simulink model "gm_whdlOFDMTx"  (R2022b)
settings: Solver=FixedStepDiscrete  StartTime=0.0  StopTime=0  RelTol=1e-3
model workspace (MATLAB code in the model file):
  | config = whdlexamples.OFDMTxParameters();
  | fftLen = config.fftLen;
  | subC = config.subC;
  | cpLen = config.cpLen;
  | fs = config.fs;
  | NSS = config.NSS;
  | NRS = config.NRS;
  | NHeader = config.NHeader;
  | NData = config.NData;
  | NSymPerF = config.NSymPerF;
  | ssSymbol = config.ssSymbol;
  | rsSymbol = config.rsSymbol;
  | NHeaderBits = config.NHeaderBits;
  | headerCRCBool = config.headerCRCBool;
  | headerConvK = config.headerConvK;
  | headerConvCode = config.headerConvCode;
  | pilotValPerSym = config.pilotValPerSym;
  | pilotLen = config.pilotLen;
  | dataCRCPoly = config.dataCRCPoly;
  | dataCRCBool = config.dataCRCBool;
  | dataCRCLen = config.dataCRCLen;
  | dataConvK = config.dataConvK;
  | dataConvCode = config.dataConvCode;
  | scramInit = config.scramInit;
  | firCoeff = config.firCoeff;
  | rateFac1 = config.rateFac1;
  | rateFac2 = config.rateFac2;
  | headerLat = config.headerLat;
  | headerTime = config.headerTime;
  | preambleInd = config.preambleInd;
  | headerDataInd = config.headerDataInd;
  | trBlkSize = config.trBlkSize;
  | randOFDM = config.randOFDM;
  | headerIntrlvMaxBlkSize = config.headerIntrlvMaxBlkSize;
  | headerIntrlvNColumns   = config.headerIntrlvNColumns;
  | dataIntrlvMaxBlkSize   = config.dataIntrlvMaxBlkSize;
  | dataIntrlvNColumns     = config.dataIntrlvNColumns;
  | clear config
libraries: hdlsllib x49, simulink x22, dspsigops x11, whdlmod x3, whdledac x3, whdlutilities x2, commhdlcrc x2, dsphdlfiltering2 x1
(part 2 of 4)

== system gm_whdlOFDMTx/Frame Controller and Input Sampler/Frame Controller/Generate Transmitter Ready ==
  valid : Inport  OutDataTypeStr=boolean  PortDimensions=1  SampleTime=4.8828125e-07
  reset : Inport  Port=2  OutDataTypeStr=boolean  PortDimensions=1  SampleTime=4.8828125e-07
  trBlkSize : Inport  Port=3  OutDataTypeStr=fixdt(0, 14, 0)  PortDimensions=1  SampleTime=4.8828125e-07
  Add : Sum  Inputs=+-  OutDataTypeStr=Inherit: Inherit via back propagation
  Compare To Constant : simulink/Logic and Bit Operations/Compare To Constant  relop===  const=0  OutDataTypeStr=boolean
  Constant : Constant  OutDataTypeStr=fixdt(0,1,0)  SampleTime=-1
  Delay : Delay  DelayLength=1
  HDL Counter : hdlsllib/Sources/HDL Counter  CountType=Count limited  CountInit=0  CountStep=1  CountMax=max(max(trBlkSize))  CountFromType=Initial value  CountFrom=0  CountResetPort=on  CountLoadPort=off  CountEnbPort=on  CountDirPort=off  CountHitOutputPort=off  CountDataType=Unsigned  CountWordLen=nextpow2(max(max(trBlkSize)) +1)  CountFracLen=0  CountSampTime=1
  Logical Operator : Logic  IconShape=distinctive  AllPortsSameDT=off  OutDataTypeStr=boolean
  Logical Operator1 : Logic  IconShape=distinctive  AllPortsSameDT=off  OutDataTypeStr=boolean
  Logical Operator2 : Logic  IconShape=distinctive  AllPortsSameDT=off  OutDataTypeStr=boolean
  Logical Operator3 : Logic  Operator=NOT  IconShape=distinctive  AllPortsSameDT=off  OutDataTypeStr=boolean
  Logical Operator4 : Logic  Operator=OR  IconShape=distinctive  AllPortsSameDT=off  OutDataTypeStr=boolean
  Relational Operator : RelationalOperator  Operator=<  OutDataTypeStr=boolean  InputSameDT=off
  Relational Operator1 : RelationalOperator  Operator===  OutDataTypeStr=boolean  InputSameDT=off
  sampleInParam : Outport  SampleTime=4.8828125e-07
  dataValid : Outport  Port=2  SampleTime=4.8828125e-07
  ready : Outport  Port=3  SampleTime=4.8828125e-07
  wires:
  valid/1 -> Logical Operator/1
  reset/1 -> HDL Counter/1
  trBlkSize/1 -> Add/1
  Add/1 -> Relational Operator1/1, Relational Operator/2
  Compare To Constant/1 -> Logical Operator1/2
  Constant/1 -> Add/2
  Delay/1 -> Logical Operator/2
  HDL Counter/1 -> Relational Operator1/2, Relational Operator/1, Compare To Constant/1
  Logical Operator/1 -> Logical Operator3/1, Logical Operator1/1, dataValid/1, HDL Counter/2
  Logical Operator1/1 -> sampleInParam/1
  Logical Operator2/1 -> Logical Operator4/2
  Logical Operator3/1 -> Logical Operator2/2
  Logical Operator4/1 -> Delay/1, ready/1
  Relational Operator/1 -> Logical Operator4/1
  Relational Operator1/1 -> Logical Operator2/1

== system gm_whdlOFDMTx/Frame Formation and OFDM Modulation/Generate OFDM Modulator Valid/Counter for Read Address ==
  enableIn : Inport  OutDataTypeStr=boolean  PortDimensions=1  SampleTime=7.8125e-06
  Counter for Read Address : MATLAB Function  TreatAsAtomicUnit=on  mask{wordLength=nextpow2(subC*NSymPerF +1), initValue=0, finalValue=subC*NSymPerF-1}
      mask prompts: wordLength "Word Length:"; initValue "Initial Value:"; finalValue "Count to value:"
  out : Outport  SampleTime=7.8125e-06  VectorParamsAs1DForOutWhenUnconnected=off
  wires:
  enableIn/1 -> Counter for Read Address/1(enableIn)
  Counter for Read Address/1(out) -> out/1

== system gm_whdlOFDMTx/Frame Formation and OFDM Modulation/Make OFDM Valid Continuous/Random OFDM Symbol ==
  in : Inport  OutDataTypeStr=boolean  PortDimensions=1  SampleTime=7.8125e-06
  Delay : Delay  DelayLength=1
  HDL Counter : hdlsllib/Sources/HDL Counter  CountType=Count limited  CountInit=0  CountStep=1  CountMax=(fftLen+cpLen) -1  CountFromType=Initial value  CountFrom=0  CountResetPort=off  CountLoadPort=off  CountEnbPort=on  CountDirPort=off  CountHitOutputPort=off  CountDataType=Unsigned  CountWordLen=nextpow2(fftLen+cpLen)  CountFracLen=0  CountSampTime=1
  Symbol LUT : Lookup_n-D  NumberOfTableDimensions=1  LookupTableObject=''  BreakpointsForDimension1=0:(length(randOFDM) -1)  BreakpointsForDimension1FirstPoint=10  BreakpointsForDimension2FirstPoint=10  BreakpointsForDimension1Spacing=12  BreakpointsForDimension2Spacing=12  IndexSearchMethod=Evenly spaced points  Table=randOFDM  InterpMethod=Flat  DiagnosticForOutOfRangeInput=Error  InternalRulePriority=Speed  OutDataTypeStr=Inherit: Inherit via back propagation  RndMeth=Simplest
  out : Outport  SampleTime=7.8125e-06  VectorParamsAs1DForOutWhenUnconnected=off
  wires:
  in/1 -> HDL Counter/1
  Delay/1 -> out/1
  HDL Counter/1 -> Symbol LUT/1
  Symbol LUT/1 -> Delay/1

== system gm_whdlOFDMTx/Frame Formation and OFDM Modulation/Make OFDM Valid Continuous/Rising Edge Detector ==
  in : Inport  OutDataTypeStr=boolean  PortDimensions=1  SampleTime=7.8125e-06
  Delay : Delay  DelayLength=1
  Logical Operator : Logic  IconShape=distinctive  AllPortsSameDT=off  OutDataTypeStr=boolean
  Logical Operator1 : Logic  Operator=NOT  IconShape=distinctive  AllPortsSameDT=off  OutDataTypeStr=boolean
  out : Outport  SampleTime=7.8125e-06
  wires:
  in/1 -> Logical Operator1/1, Logical Operator/1
  Delay/1 -> Logical Operator/2
  Logical Operator/1 -> out/1
  Logical Operator1/1 -> Delay/1

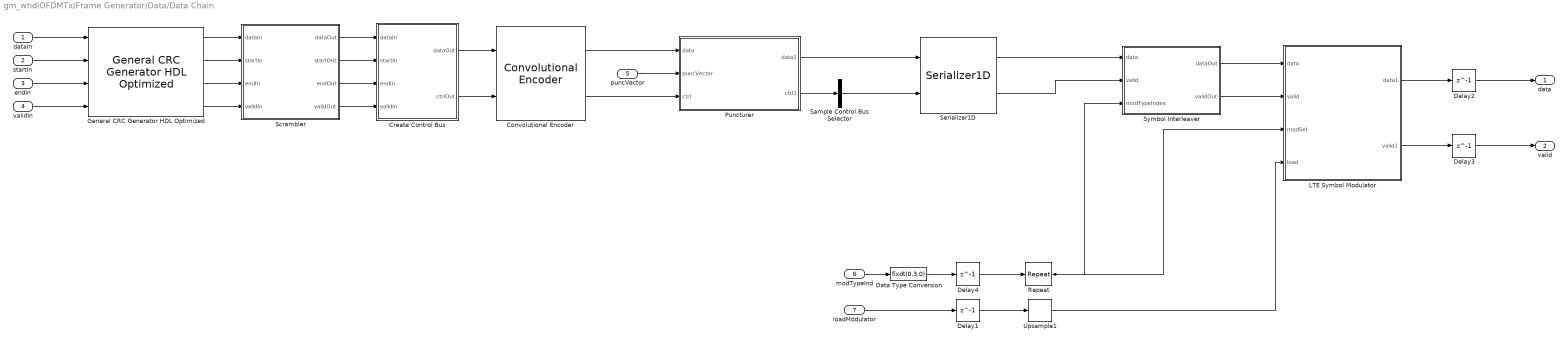
== system gm_whdlOFDMTx/Frame Generator/Data/Data Chain ==
  dataIn : Inport  OutDataTypeStr=boolean  PortDimensions=1  SampleTime=4.8828125e-07
  startIn : Inport  Port=2  OutDataTypeStr=boolean  PortDimensions=1  SampleTime=4.8828125e-07
  endIn : Inport  Port=3  OutDataTypeStr=boolean  PortDimensions=1  SampleTime=4.8828125e-07
  validIn : Inport  Port=4  OutDataTypeStr=boolean  PortDimensions=1  SampleTime=4.8828125e-07
  puncVector : Inport  Port=5  OutDataTypeStr=boolean  PortDimensions=[10]  SampleTime=4.8828125e-07
  modTypeInd : Inport  Port=6  OutDataTypeStr=fixdt(0, 2, 0)  PortDimensions=1  SampleTime=4.8828125e-07
  loadModulator : Inport  Port=7  OutDataTypeStr=boolean  PortDimensions=1  SampleTime=4.8828125e-07
  Convolutional Encoder : whdledac/Convolutional Encoder  ConstraintLength=dataConvK  CodeGenerator=dataConvCode  FeedbackConnection=0  TerminationMethod=Terminated  ResetPort=off  InitialStatePort=off  FinalStatePort=off  SimulateUsing=Code generation
  Create Control Bus : Subsystem
  Data Type Conversion : DataTypeConversion  OutDataTypeStr=fixdt(0,3,0)  SaturateOnIntegerOverflow=off  RndMeth=Floor
  Delay{1..4} (4 alike) : Delay  DelayLength=1
  General CRC Generator HDL Optimized : commhdlcrc/General CRC Generator HDL Optimized  Polynomial=dataCRCBool  InitialState=0  DirectMethod=off  ReflectInput=off  ReflectCRCChecksum=off  FinalXORValue=0  SimulateUsing=Code generation
  LTE Symbol Modulator : Subsystem
  Puncturer : Subsystem
  Repeat : dspsigops/Repeat  N=length(dataConvCode)  RateOptions=Allow multirate processing  ic=0  mode=Unused parameter value
  Sample Control Bus Selector : BusSelector  OutputSignals=valid
  Scrambler : Subsystem
  Serializer1D : hdlsllib/HDL Operations/Serializer1D  Ratio=length(dataConvCode)/1  IdleCycles=0  validIn=on  startOut=off  validOut=on  inputDataDimensions=-1  inputSampleTime=-1  inputSignalType=auto
  Symbol Interleaver : Subsystem
  Upsample1 : dspsigops/Upsample  N=length(dataConvCode)  phase=0  RateOptions=Allow multirate processing  ic=0  mode=Unused parameter value
  data : Outport  SampleTime=2.44140625e-07
  valid : Outport  Port=2  SampleTime=2.44140625e-07
  wires:
  dataIn/1 -> General CRC Generator HDL Optimized/1
  startIn/1 -> General CRC Generator HDL Optimized/2
  endIn/1 -> General CRC Generator HDL Optimized/3
  validIn/1 -> General CRC Generator HDL Optimized/4
  puncVector/1 -> Puncturer/2(puncVector)
  modTypeInd/1 -> Data Type Conversion/1
  loadModulator/1 -> Delay1/1
  Convolutional Encoder/1 -> Puncturer/1(data)
  Convolutional Encoder/2 -> Puncturer/3(ctrl)
  Create Control Bus/1(dataOut) -> Convolutional Encoder/1
  Create Control Bus/2(ctrlOut) -> Convolutional Encoder/2
  Data Type Conversion/1 -> Delay4/1
  Delay1/1 -> Upsample1/1
  Delay2/1 -> data/1
  Delay3/1 -> valid/1
  Delay4/1 -> Repeat/1
  General CRC Generator HDL Optimized/1 -> Scrambler/1(dataIn)
  General CRC Generator HDL Optimized/2 -> Scrambler/2(startIn)
  General CRC Generator HDL Optimized/3 -> Scrambler/3(endIn)
  General CRC Generator HDL Optimized/4 -> Scrambler/4(validIn)
  LTE Symbol Modulator/1(data1) -> Delay2/1
  LTE Symbol Modulator/2(valid1) -> Delay3/1
  Puncturer/1(data1) -> Serializer1D/1
  Puncturer/2(ctrl1) -> Sample Control Bus Selector/1
  Repeat/1 -> LTE Symbol Modulator/3(modSel), Symbol Interleaver/3(modTypeIndex)
  Sample Control Bus Selector/1 -> Serializer1D/2
  Scrambler/1(dataOut) -> Create Control Bus/1(dataIn)
  Scrambler/2(startOut) -> Create Control Bus/2(startIn)
  Scrambler/3(endOut) -> Create Control Bus/3(endIn)
  Scrambler/4(validOut) -> Create Control Bus/4(validIn)
  Serializer1D/1 -> Symbol Interleaver/1(data)
  Serializer1D/2 -> Symbol Interleaver/2(valid)
  Symbol Interleaver/1(dataOut) -> LTE Symbol Modulator/1(data)
  Symbol Interleaver/2(validOut) -> LTE Symbol Modulator/2(valid)
  Upsample1/1 -> LTE Symbol Modulator/4(load)

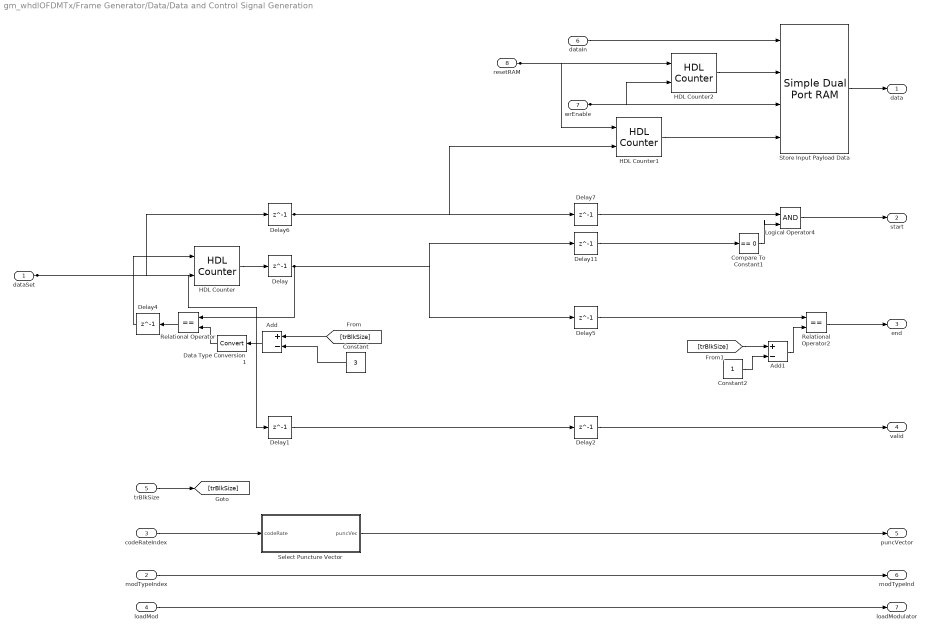
== system gm_whdlOFDMTx/Frame Generator/Data/Data and Control Signal Generation ==
  dataSet : Inport  OutDataTypeStr=boolean  PortDimensions=1  SampleTime=4.8828125e-07
  modTypeIndex : Inport  Port=2  OutDataTypeStr=fixdt(0, 2, 0)  PortDimensions=1  SampleTime=4.8828125e-07
  codeRateIndex : Inport  Port=3  OutDataTypeStr=fixdt(0, 2, 0)  PortDimensions=1  SampleTime=4.8828125e-07
  loadMod : Inport  Port=4  OutDataTypeStr=boolean  PortDimensions=1  SampleTime=4.8828125e-07
  trBlkSize : Inport  Port=5  OutDataTypeStr=fixdt(0, 14, 0)  PortDimensions=1  SampleTime=4.8828125e-07
  dataIn : Inport  Port=6  OutDataTypeStr=boolean  PortDimensions=1  SampleTime=4.8828125e-07
  wrEnable : Inport  Port=7  OutDataTypeStr=boolean  PortDimensions=1  SampleTime=4.8828125e-07
  resetRAM : Inport  Port=8  OutDataTypeStr=boolean  PortDimensions=1  SampleTime=4.8828125e-07
  Add : Sum  Inputs=+-
  Add1 : Sum  Inputs=+-  OutDataTypeStr=Inherit: Same as first input
  Compare To Constant1 : simulink/Logic and Bit Operations/Compare To Constant  relop===  const=0  OutDataTypeStr=boolean
  Constant : Constant  Value=3  OutDataTypeStr=Inherit: Inherit via back propagation  SampleTime=-1
  Constant2 : Constant  OutDataTypeStr=Inherit: Inherit via back propagation  SampleTime=-1
  Data Type Conversion1 : DataTypeConversion  SaturateOnIntegerOverflow=off  RndMeth=Floor
  Delay{,1..2,4..7,11} (8 alike) : Delay  DelayLength=1
  HDL Counter : hdlsllib/Sources/HDL Counter  CountType=Count limited  CountInit=0  CountStep=1  CountMax=max(max(trBlkSize)) - 1  CountFromType=Initial value  CountFrom=0  CountResetPort=on  CountLoadPort=off  CountEnbPort=on  CountDirPort=off  CountHitOutputPort=off  CountDataType=Unsigned  CountWordLen=nextpow2(max(max(trBlkSize)) - 1 +1)  CountFracLen=0  CountSampTime=1
  HDL Counter1 : hdlsllib/Sources/HDL Counter  CountType=Count limited  CountInit=0  CountStep=1  CountMax=max(max(trBlkSize)) -1  CountFromType=Initial value  CountFrom=0  CountResetPort=on  CountLoadPort=off  CountEnbPort=on  CountDirPort=off  CountHitOutputPort=off  CountDataType=Unsigned  CountWordLen=nextpow2(max(max(trBlkSize)) -1 +1)  CountFracLen=0  CountSampTime=1
  HDL Counter2 : hdlsllib/Sources/HDL Counter  CountType=Count limited  CountInit=0  CountStep=1  CountMax=max(max(trBlkSize))  CountFromType=Initial value  CountFrom=0  CountResetPort=on  CountLoadPort=off  CountEnbPort=on  CountDirPort=off  CountHitOutputPort=off  CountDataType=Unsigned  CountWordLen=nextpow2(max(max(trBlkSize)) +1)  CountFracLen=0  CountSampTime=1
  Logical Operator4 : Logic  IconShape=distinctive  AllPortsSameDT=off  OutDataTypeStr=boolean
  Relational Operator : RelationalOperator  Operator===  OutDataTypeStr=boolean  InputSameDT=off
  Relational Operator2 : RelationalOperator  Operator===  OutDataTypeStr=boolean  InputSameDT=off
  Select Puncture Vector : Subsystem
  Store Input Payload Data : hdlsllib/HDL RAMs/Simple Dual Port RAM  ram_size=nextpow2(max(max(trBlkSize)) +1)
  data : Outport  SampleTime=4.8828125e-07
  start : Outport  Port=2  SampleTime=4.8828125e-07
  end : Outport  Port=3  SampleTime=4.8828125e-07
  valid : Outport  Port=4  SampleTime=4.8828125e-07
  puncVector : Outport  Port=5  SampleTime=4.8828125e-07
  modTypeInd : Outport  Port=6  SampleTime=4.8828125e-07
  loadModulator : Outport  Port=7  SampleTime=4.8828125e-07
  wires:
  dataSet/1 -> Delay6/1, Delay1/1, HDL Counter/2
  modTypeIndex/1 -> modTypeInd/1
  codeRateIndex/1 -> Select Puncture Vector/1(codeRate)
  loadMod/1 -> loadModulator/1
  trBlkSize/1 -> [trBlkSize]
  dataIn/1 -> Store Input Payload Data/1
  wrEnable/1 -> Store Input Payload Data/3, HDL Counter2/2
  resetRAM/1 -> HDL Counter1/1, HDL Counter2/1
  Add/1 -> Data Type Conversion1/1
  Add1/1 -> Relational Operator2/2
  Compare To Constant1/1 -> Logical Operator4/2
  Constant/1 -> Add/2
  Constant2/1 -> Add1/2
  Data Type Conversion1/1 -> Relational Operator/2
  Delay/1 -> Relational Operator/1, Delay5/1, Delay11/1
  Delay1/1 -> Delay2/1
  Delay11/1 -> Compare To Constant1/1
  Delay2/1 -> valid/1
  Delay4/1 -> HDL Counter/1
  Delay5/1 -> Relational Operator2/1
  Delay6/1 -> Delay7/1, HDL Counter1/2
  Delay7/1 -> Logical Operator4/1
  [trBlkSize] -> Add/1
  [trBlkSize] -> Add1/1
  HDL Counter/1 -> Delay/1
  HDL Counter1/1 -> Store Input Payload Data/4
  HDL Counter2/1 -> Store Input Payload Data/2
  Logical Operator4/1 -> start/1
  Relational Operator/1 -> Delay4/1
  Relational Operator2/1 -> end/1
  Select Puncture Vector/1(puncVec) -> puncVector/1
  Store Input Payload Data/1 -> data/1

== system gm_whdlOFDMTx/Frame Generator/Header/Create Control Bus ==
  dataIn : Inport  OutDataTypeStr=boolean  PortDimensions=1  SampleTime=4.8828125e-07
  startIn : Inport  Port=2  OutDataTypeStr=boolean  PortDimensions=1  SampleTime=4.8828125e-07
  endIn : Inport  Port=3  OutDataTypeStr=boolean  PortDimensions=1  SampleTime=4.8828125e-07
  validIn : Inport  Port=4  OutDataTypeStr=boolean  PortDimensions=1  SampleTime=4.8828125e-07
  Sample Control Bus Creator : whdlutilities/Sample Control Bus Creator
  dataOut : Outport  SampleTime=4.8828125e-07
  ctrlOut : Outport  Port=2
  wires:
  dataIn/1 -> dataOut/1
  startIn/1 -> Sample Control Bus Creator/1
  endIn/1 -> Sample Control Bus Creator/2
  validIn/1 -> Sample Control Bus Creator/3
  Sample Control Bus Creator/1 -> ctrlOut/1

== system gm_whdlOFDMTx/Frame Generator/Header/Header Formation ==
  modType : Inport  OutDataTypeStr=fixdt(0, 2, 0)  PortDimensions=1  SampleTime=4.8828125e-07
  codeRate : Inport  Port=2  OutDataTypeStr=fixdt(0, 2, 0)  PortDimensions=1  SampleTime=4.8828125e-07
  fftLen : Inport  Port=3  OutDataTypeStr=fixdt(0, 3, 0)  PortDimensions=1  SampleTime=4.8828125e-07
  validIn : Inport  Port=4  OutDataTypeStr=boolean  PortDimensions=1  SampleTime=4.8828125e-07
  Header Formation : MATLAB Function  TreatAsAtomicUnit=on  mask{NHeaderBits=NHeaderBits}
      mask prompts: NHeaderBits "Number of Header Bits:"
  headerBits : Outport  SampleTime=4.8828125e-07  VectorParamsAs1DForOutWhenUnconnected=off
  startOut : Outport  Port=2  SampleTime=4.8828125e-07
  endOut : Outport  Port=3  SampleTime=4.8828125e-07
  validOut : Outport  Port=4  SampleTime=4.8828125e-07
  wires:
  modType/1 -> Header Formation/1(modType)
  codeRate/1 -> Header Formation/2(codeRate)
  fftLen/1 -> Header Formation/3(fftLen)
  validIn/1 -> Header Formation/4(validIn)
  Header Formation/1(headerBits) -> headerBits/1
  Header Formation/2(startOut) -> startOut/1
  Header Formation/3(endOut) -> endOut/1
  Header Formation/4(validOut) -> validOut/1

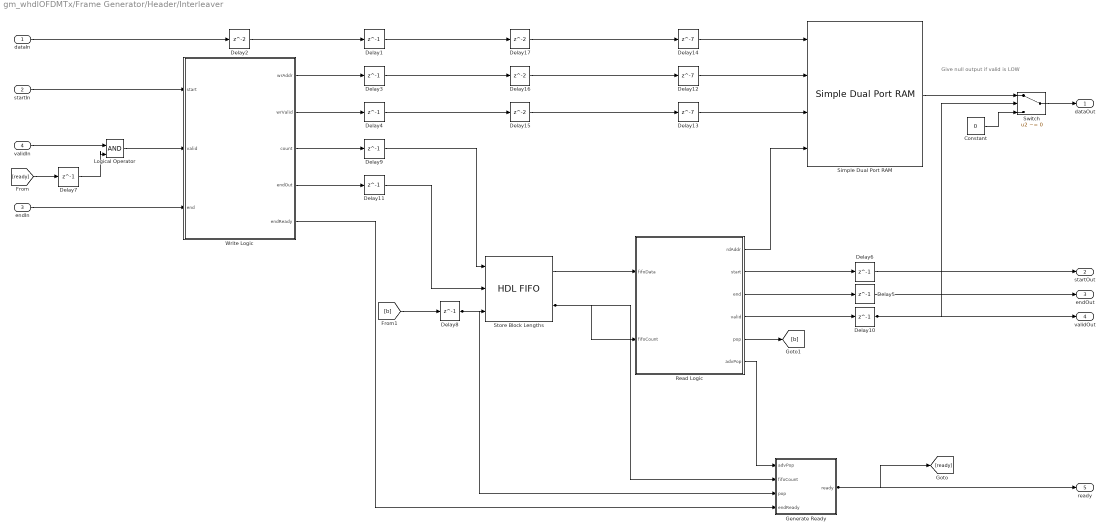
== system gm_whdlOFDMTx/Frame Generator/Header/Interleaver ==
  note: Give null output if valid is LOW
  dataIn : Inport  OutDataTypeStr=boolean  PortDimensions=1  SampleTime=2.44140625e-07
  startIn : Inport  Port=2  OutDataTypeStr=boolean  PortDimensions=1  SampleTime=2.44140625e-07
  endIn : Inport  Port=3  OutDataTypeStr=boolean  PortDimensions=1  SampleTime=2.44140625e-07
  validIn : Inport  Port=4  OutDataTypeStr=boolean  PortDimensions=1  SampleTime=2.44140625e-07
  Constant : Constant  Value=0  OutDataTypeStr=Inherit: Inherit via back propagation  SampleTime=-1
  Delay{1,3..6,9..11} (8 alike) : Delay  DelayLength=1
  Delay12 : Delay  DelayLength=7
  Delay13 : Delay  DelayLength=7
  Delay14 : Delay  DelayLength=7
  Delay{2,15..17} (4 alike) : Delay
  Delay7 : Delay  DelayLength=1  InitialCondition=true
  Delay8 : Delay  DelayLength=1  InitialCondition=true
  Generate Ready : Subsystem
  Logical Operator : Logic  IconShape=distinctive  AllPortsSameDT=off  OutDataTypeStr=boolean
  Read Logic : Subsystem
  Simple Dual Port RAM : hdlsllib/HDL RAMs/Simple Dual Port RAM  ram_size=nextpow2(2*maxBlkSize)
  Store Block Lengths : hdlsllib/HDL RAMs/HDL FIFO  fifo_size=4  mode=Classic  ratio=1  push_msg=Warning  pop_msg=Ignore  show_empty=off  show_full=off  show_num=on  LabelModeActiveChoice_Mode=Classic  rst_port=off
  Switch : Switch  Criteria=u2 ~= 0  SaturateOnIntegerOverflow=off
  Write Logic : Subsystem
  dataOut : Outport  SampleTime=2.44140625e-07
  startOut : Outport  Port=2  SampleTime=2.44140625e-07
  endOut : Outport  Port=3  SampleTime=2.44140625e-07
  validOut : Outport  Port=4  SampleTime=2.44140625e-07
  ready : Outport  Port=5  SampleTime=2.44140625e-07
  wires:
  dataIn/1 -> Delay2/1
  startIn/1 -> Write Logic/1(start)
  endIn/1 -> Write Logic/3(end)
  validIn/1 -> Logical Operator/1
  Constant/1 -> Switch/3
  Delay1/1 -> Delay17/1
  Delay10/1 -> Switch/2, validOut/1
  Delay11/1 -> Store Block Lengths/2
  Delay12/1 -> Simple Dual Port RAM/2
  Delay13/1 -> Simple Dual Port RAM/3
  Delay14/1 -> Simple Dual Port RAM/1
  Delay15/1 -> Delay13/1
  Delay16/1 -> Delay12/1
  Delay17/1 -> Delay14/1
  Delay2/1 -> Delay1/1
  Delay3/1 -> Delay16/1
  Delay4/1 -> Delay15/1
  Delay5/1 -> endOut/1
  Delay6/1 -> startOut/1
  Delay7/1 -> Logical Operator/2
  Delay8/1 -> Generate Ready/3(pop), Store Block Lengths/3
  Delay9/1 -> Store Block Lengths/1
  [ready] -> Delay7/1
  [b] -> Delay8/1
  Generate Ready/1(ready) -> [ready], ready/1
  Logical Operator/1 -> Write Logic/2(valid)
  Read Logic/1(rdAddr) -> Simple Dual Port RAM/4
  Read Logic/2(start) -> Delay6/1
  Read Logic/3(end) -> Delay5/1
  Read Logic/4(valid) -> Delay10/1
  Read Logic/5(pop) -> [b]
  Read Logic/6(advPop) -> Generate Ready/1(advPop)
  Simple Dual Port RAM/1 -> Switch/1
  Store Block Lengths/1 -> Read Logic/1(fifoData)
  Store Block Lengths/2 -> Generate Ready/2(fifoCount), Read Logic/2(fifoCount)
  Switch/1 -> dataOut/1
  Write Logic/1(wrAddr) -> Delay3/1
  Write Logic/2(wrValid) -> Delay4/1
  Write Logic/3(count) -> Delay9/1
  Write Logic/4(endOut) -> Delay11/1
  Write Logic/5(endReady) -> Generate Ready/4(endReady)

== system gm_whdlOFDMTx/Frame Generator/Header/LTE Symbol Modulator ==
  data : Inport  OutDataTypeStr=boolean  SampleTime=2.44140625e-07
  valid : Inport  Port=2  OutDataTypeStr=boolean  SampleTime=2.44140625e-07
  LTE Symbol Modulator : whdlmod/LTE Symbol Modulator  ModulationSource=Property  ModulationScheme=BPSK  SimulateUsing=Code generation  OutputDataType=Custom  WordLength=16
  data1 : Outport  SampleTime=2.44140625e-07
  valid1 : Outport  Port=2  SampleTime=2.44140625e-07
  wires:
  data/1 -> LTE Symbol Modulator/1
  valid/1 -> LTE Symbol Modulator/2
  LTE Symbol Modulator/1 -> data1/1
  LTE Symbol Modulator/2 -> valid1/1

== system gm_whdlOFDMTx/Frame Generator/Header/Serializer ==
  parallelIn : Inport  OutDataTypeStr=boolean  PortDimensions=[2 1]  SampleTime=4.8828125e-07
  ctrlIn : Inport  Port=2
  Delay : Delay  DelayLength=1
  Delay1 : Delay  DelayLength=1
  Sample Control Bus Selector : BusSelector  OutputSignals=valid,start,end
  Serialize Start and End Signals : Subsystem
  Serializer1D : hdlsllib/HDL Operations/Serializer1D  Ratio=length(headerConvCode)/1  IdleCycles=0  validIn=on  startOut=off  validOut=on  inputDataDimensions=-1  inputSampleTime=-1  inputSignalType=auto
  serialOut : Outport  SampleTime=2.44140625e-07
  startOut : Outport  Port=2  SampleTime=2.44140625e-07
  endOut : Outport  Port=3  SampleTime=2.44140625e-07
  ValidOut : Outport  Port=4  SampleTime=2.44140625e-07
  wires:
  parallelIn/1 -> Serializer1D/1
  ctrlIn/1 -> Sample Control Bus Selector/1
  Delay/1 -> ValidOut/1
  Delay1/1 -> serialOut/1
  Sample Control Bus Selector/1 -> Serializer1D/2
  Sample Control Bus Selector/2 -> Serialize Start and End Signals/1(startIn)
  Sample Control Bus Selector/3 -> Serialize Start and End Signals/2(endIn)
  Serialize Start and End Signals/1(startOut) -> startOut/1
  Serialize Start and End Signals/2(endOut) -> endOut/1
  Serializer1D/1 -> Delay1/1
  Serializer1D/2 -> Delay/1

== system gm_whdlOFDMTx/Multiplexer/Multiplex Preamble Signals/Priority Encoder ==
  ssValid : Inport  OutDataTypeStr=boolean  PortDimensions=1  SampleTime=2.44140625e-07
  rsValid : Inport  Port=2  OutDataTypeStr=boolean  PortDimensions=1  SampleTime=2.44140625e-07
  pilotValid : Inport  Port=3  OutDataTypeStr=boolean  PortDimensions=1  SampleTime=2.44140625e-07
  Priority Encoder : MATLAB Function  TreatAsAtomicUnit=on
  selLine : Outport  SampleTime=2.44140625e-07  VectorParamsAs1DForOutWhenUnconnected=off
  wires:
  ssValid/1 -> Priority Encoder/1(ssValid)
  rsValid/1 -> Priority Encoder/2(rsValid)
  pilotValid/1 -> Priority Encoder/3(pilotValid)
  Priority Encoder/1(selLine) -> selLine/1

== system gm_whdlOFDMTx/Frame Controller and Input Sampler/Frame Controller/Generate OFDM Modulator Ready/Control OFDM Signal Generation ==
  readyLow : Inport  OutDataTypeStr=boolean  PortDimensions=1  SampleTime=4.8828125e-07
  reset : Inport  Port=2  OutDataTypeStr=boolean  PortDimensions=1  SampleTime=4.8828125e-07
  Disable OFDM Generation : Subsystem
  Falling Edge Detector : Subsystem
  Logical Operator11 : Logic  Operator=OR  Inputs=3  IconShape=distinctive  AllPortsSameDT=off  OutDataTypeStr=boolean
  Logical Operator6 : Logic  Operator=OR  IconShape=distinctive  AllPortsSameDT=off  OutDataTypeStr=boolean
  Logical Operator8 : Logic  Operator=NOT  IconShape=distinctive  AllPortsSameDT=off  OutDataTypeStr=boolean
  MATLAB Function2 : Subsystem
  Pulse Generator : Subsystem
  holdOFDMGen : Outport  SampleTime=4.8828125e-07
  wires:
  readyLow/1 -> Disable OFDM Generation/1(readyLow)
  reset/1 -> Logical Operator6/2
  Disable OFDM Generation/1(out) -> Logical Operator11/1
  Falling Edge Detector/1(out) -> Logical Operator11/2, Disable OFDM Generation/2(waitSignal)
  Logical Operator11/1 -> Logical Operator8/1
  Logical Operator6/1 -> MATLAB Function2/1(trigger)
  Logical Operator8/1 -> holdOFDMGen/1
  MATLAB Function2/1(out) -> Logical Operator11/3, Falling Edge Detector/1(in)
  Pulse Generator/1(pulse) -> Logical Operator6/1

== system gm_whdlOFDMTx/Frame Controller and Input Sampler/Frame Controller/Generate OFDM Modulator Ready/MATLAB Function1 ==
  trigger : Inport  OutDataTypeStr=boolean  PortDimensions=1  SampleTime=4.8828125e-07
  MATLAB Function1 : MATLAB Function  TreatAsAtomicUnit=on  mask{nClocks=(NSymPerF*(fftLen+cpLen))*rateFac2}
      mask prompts: nClocks "Number of clocks to hold:"
  out : Outport  SampleTime=4.8828125e-07  VectorParamsAs1DForOutWhenUnconnected=off
  wires:
  trigger/1 -> MATLAB Function1/1(trigger)
  MATLAB Function1/1(out) -> out/1

== system gm_whdlOFDMTx/Frame Controller and Input Sampler/Frame Controller/Generate OFDM Modulator Ready/Rising Edge Detector ==
  in : Inport  OutDataTypeStr=boolean  PortDimensions=1  SampleTime=4.8828125e-07
  Delay : Delay  DelayLength=1
  Logical Operator1 : Logic  IconShape=distinctive  AllPortsSameDT=off  OutDataTypeStr=boolean
  Logical Operator2 : Logic  Operator=NOT  IconShape=distinctive  AllPortsSameDT=off  OutDataTypeStr=boolean
  out : Outport  SampleTime=4.8828125e-07
  wires:
  in/1 -> Logical Operator2/1, Logical Operator1/2
  Delay/1 -> Logical Operator1/1
  Logical Operator1/1 -> out/1
  Logical Operator2/1 -> Delay/1

== system gm_whdlOFDMTx/Frame Generator/Data/Data Chain/Create Control Bus ==
  dataIn : Inport  OutDataTypeStr=boolean  PortDimensions=1  SampleTime=4.8828125e-07
  startIn : Inport  Port=2  OutDataTypeStr=boolean  PortDimensions=1  SampleTime=4.8828125e-07
  endIn : Inport  Port=3  OutDataTypeStr=boolean  PortDimensions=1  SampleTime=4.8828125e-07
  validIn : Inport  Port=4  OutDataTypeStr=boolean  PortDimensions=1  SampleTime=4.8828125e-07
  Sample Control Bus Creator : whdlutilities/Sample Control Bus Creator
  dataOut : Outport  SampleTime=4.8828125e-07
  ctrlOut : Outport  Port=2
  wires:
  dataIn/1 -> dataOut/1
  startIn/1 -> Sample Control Bus Creator/1
  endIn/1 -> Sample Control Bus Creator/2
  validIn/1 -> Sample Control Bus Creator/3
  Sample Control Bus Creator/1 -> ctrlOut/1

== system gm_whdlOFDMTx/Frame Generator/Data/Data Chain/LTE Symbol Modulator ==
  data : Inport  OutDataTypeStr=boolean  SampleTime=2.44140625e-07
  valid : Inport  Port=2  OutDataTypeStr=boolean  SampleTime=2.44140625e-07
  modSel : Inport  Port=3  OutDataTypeStr=fixdt(0, 3, 0)  SampleTime=2.44140625e-07
  load : Inport  Port=4  OutDataTypeStr=boolean  SampleTime=2.44140625e-07
  LTE Symbol Modulator : whdlmod/LTE Symbol Modulator  ModulationSource=Input port  ModulationScheme=BPSK  SimulateUsing=Code generation  OutputDataType=Custom  WordLength=16
  data1 : Outport  SampleTime=2.44140625e-07
  valid1 : Outport  Port=2  SampleTime=2.44140625e-07
  wires:
  data/1 -> LTE Symbol Modulator/1
  valid/1 -> LTE Symbol Modulator/2
  modSel/1 -> LTE Symbol Modulator/3
  load/1 -> LTE Symbol Modulator/4
  LTE Symbol Modulator/1 -> data1/1
  LTE Symbol Modulator/2 -> valid1/1

== system gm_whdlOFDMTx/Frame Generator/Data/Data Chain/Puncturer ==
  data : Inport  OutDataTypeStr=boolean  PortDimensions=[2 1]  SampleTime=4.8828125e-07
  puncVector : Inport  Port=2  OutDataTypeStr=boolean  PortDimensions=[10]  SampleTime=4.8828125e-07
  ctrl : Inport  Port=3  SampleTime=4.8828125e-07
  Puncturer : whdledac/Puncturer  OpMode=Frame  EncRate=1/2  VecSource=Input port  puncVector=[1;1;1;0;0;1]  SimulateUsing=Code generation
  data1 : Outport  SampleTime=4.8828125e-07
  ctrl1 : Outport  Port=2  SampleTime=4.8828125e-07
  wires:
  data/1 -> Puncturer/1
  puncVector/1 -> Puncturer/2
  ctrl/1 -> Puncturer/3
  Puncturer/1 -> data1/1
  Puncturer/2 -> ctrl1/1

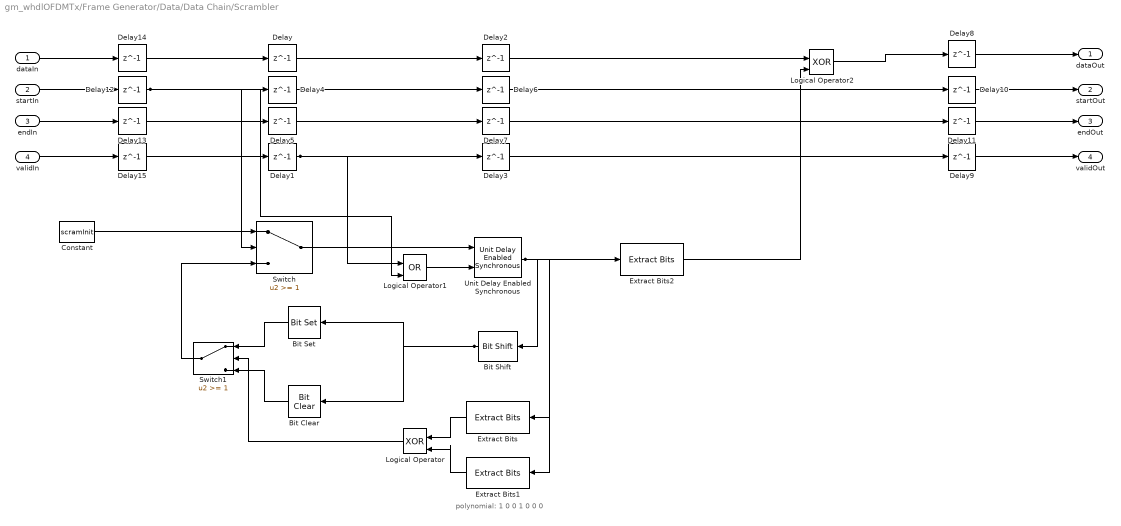
== system gm_whdlOFDMTx/Frame Generator/Data/Data Chain/Scrambler ==
  note: polynomial: 1 0 0 1 0 0 0
  dataIn : Inport  OutDataTypeStr=boolean  PortDimensions=1  SampleTime=4.8828125e-07
  startIn : Inport  Port=2  OutDataTypeStr=boolean  PortDimensions=1  SampleTime=4.8828125e-07
  endIn : Inport  Port=3  OutDataTypeStr=boolean  PortDimensions=1  SampleTime=4.8828125e-07
  validIn : Inport  Port=4  OutDataTypeStr=boolean  PortDimensions=1  SampleTime=4.8828125e-07
  Bit Clear : simulink/Logic and Bit Operations/Bit Clear  iBit=0
  Bit Set : simulink/Logic and Bit Operations/Bit Set  iBit=0
  Bit Shift : hdlsllib/Logic and Bit Operations/Bit Shift  mode=Shift Left Logical  N=1
  Constant : Constant  Value=scramInit  OutDataTypeStr=fixdt(0,7,0)  SampleTime=-1
  Delay{,1..15} (16 alike) : Delay  DelayLength=1
  Extract Bits : simulink/Logic and Bit Operations/Extract Bits  bitsToExtract=Range of bits  numBits=8  bitIdxRange=3  outScalingMode=Preserve fixed-point scaling
  Extract Bits1 : simulink/Logic and Bit Operations/Extract Bits  bitsToExtract=Range of bits  numBits=8  bitIdxRange=6  outScalingMode=Preserve fixed-point scaling
  Extract Bits2 : simulink/Logic and Bit Operations/Extract Bits  bitsToExtract=Range of bits  numBits=8  bitIdxRange=0  outScalingMode=Preserve fixed-point scaling
  Logical Operator : Logic  Operator=XOR  IconShape=distinctive  AllPortsSameDT=off  OutDataTypeStr=boolean
  Logical Operator1 : Logic  Operator=OR  IconShape=distinctive  AllPortsSameDT=off  OutDataTypeStr=boolean
  Logical Operator2 : Logic  Operator=XOR  IconShape=distinctive  AllPortsSameDT=off  OutDataTypeStr=boolean
  Switch : Switch  Threshold=1  SaturateOnIntegerOverflow=off  InputSameDT=off
  Switch1 : Switch  Threshold=1  SaturateOnIntegerOverflow=off  InputSameDT=off
  Unit Delay Enabled Synchronous : hdlsllib/Discrete/Unit Delay Enabled Synchronous  InitialCondition=0.0  SampleTime=-1
  dataOut : Outport  SampleTime=4.8828125e-07
  startOut : Outport  Port=2  SampleTime=4.8828125e-07
  endOut : Outport  Port=3  SampleTime=4.8828125e-07
  validOut : Outport  Port=4  SampleTime=4.8828125e-07
  wires:
  dataIn/1 -> Delay14/1
  startIn/1 -> Delay12/1
  endIn/1 -> Delay13/1
  validIn/1 -> Delay15/1
  Bit Clear/1 -> Switch1/3
  Bit Set/1 -> Switch1/1
  Bit Shift/1 -> Bit Set/1, Bit Clear/1
  Constant/1 -> Switch/1
  Delay/1 -> Delay2/1
  Delay1/1 -> Logical Operator1/1, Delay3/1
  Delay10/1 -> startOut/1
  Delay11/1 -> endOut/1
  Delay12/1 -> Switch/2, Logical Operator1/2, Delay4/1
  Delay13/1 -> Delay5/1
  Delay14/1 -> Delay/1
  Delay15/1 -> Delay1/1
  Delay2/1 -> Logical Operator2/1
  Delay3/1 -> Delay9/1
  Delay4/1 -> Delay6/1
  Delay5/1 -> Delay7/1
  Delay6/1 -> Delay10/1
  Delay7/1 -> Delay11/1
  Delay8/1 -> dataOut/1
  Delay9/1 -> validOut/1
  Extract Bits/1 -> Logical Operator/1
  Extract Bits1/1 -> Logical Operator/2
  Extract Bits2/1 -> Logical Operator2/2
  Logical Operator/1 -> Switch1/2
  Logical Operator1/1 -> Unit Delay Enabled Synchronous/2
  Logical Operator2/1 -> Delay8/1
  Switch/1 -> Unit Delay Enabled Synchronous/1
  Switch1/1 -> Switch/3
  Unit Delay Enabled Synchronous/1 -> Extract Bits2/1, Extract Bits1/1, Extract Bits/1, Bit Shift/1

== system gm_whdlOFDMTx/Frame Generator/Data/Data Chain/Symbol Interleaver ==
  data : Inport  OutDataTypeStr=boolean  PortDimensions=1  SampleTime=2.44140625e-07
  valid : Inport  Port=2  OutDataTypeStr=boolean  PortDimensions=1  SampleTime=2.44140625e-07
  modTypeIndex : Inport  Port=3  OutDataTypeStr=fixdt(0, 3, 0)  PortDimensions=1  SampleTime=2.44140625e-07
  Interleaver : Subsystem  mask{maxBlkSize=double(360), nColumns=double(15)}
      mask prompts: maxBlkSize "Maximum block size:"; nColumns "Number of columns:"
      mask init:
      | maxBlkSize = double(360);
      | maxNRows = double(24);
      | nColumns = double(15);
  Interleaver_term1 : Terminator
  Interleaver_term2 : Terminator
  Interleaver_term4 : Terminator
  Split Data Into Symbols : Subsystem
  dataOut : Outport  SampleTime=2.44140625e-07
  validOut : Outport  Port=2  SampleTime=2.44140625e-07
  wires:
  data/1 -> Split Data Into Symbols/1(data)
  valid/1 -> Split Data Into Symbols/2(valid)
  modTypeIndex/1 -> Split Data Into Symbols/3(modTypeIndex)
  Interleaver/1(dataOut) -> dataOut/1
  Interleaver/2(startOut) -> Interleaver_term1/1
  Interleaver/3(endOut) -> Interleaver_term2/1
  Interleaver/4(validOut) -> validOut/1
  Interleaver/5(ready) -> Interleaver_term4/1
  Split Data Into Symbols/1(dataOut) -> Interleaver/1(dataIn)
  Split Data Into Symbols/2(startOut) -> Interleaver/2(startIn)
  Split Data Into Symbols/3(endOut) -> Interleaver/3(endIn)
  Split Data Into Symbols/4(validOut) -> Interleaver/4(validIn)

== system gm_whdlOFDMTx/Frame Generator/Data/Data and Control Signal Generation/Select Puncture Vector ==
  codeRate : Inport  OutDataTypeStr=fixdt(0, 2, 0)  PortDimensions=1  SampleTime=4.8828125e-07
  Select Puncture Vector : MATLAB Function  TreatAsAtomicUnit=on
  puncVec : Outport  SampleTime=4.8828125e-07  VectorParamsAs1DForOutWhenUnconnected=off
  wires:
  codeRate/1 -> Select Puncture Vector/1(codeRate)
  Select Puncture Vector/1(puncVec) -> puncVec/1

== system gm_whdlOFDMTx/Frame Generator/Header/Interleaver/Generate Ready ==
  advPop : Inport  OutDataTypeStr=boolean  PortDimensions=1  SampleTime=2.44140625e-07
  fifoCount : Inport  Port=2  OutDataTypeStr=fixdt(0, 3, 0)  PortDimensions=1  SampleTime=2.44140625e-07
  pop : Inport  Port=3  OutDataTypeStr=boolean  PortDimensions=1  SampleTime=2.44140625e-07
  endReady : Inport  Port=4  OutDataTypeStr=boolean  PortDimensions=1  SampleTime=2.44140625e-07
  Generate Ready2 : Subsystem
  Logical Operator1 : Logic  IconShape=distinctive  AllPortsSameDT=off  OutDataTypeStr=boolean
  Logical Operator2 : Logic  IconShape=distinctive  AllPortsSameDT=off  OutDataTypeStr=boolean
  Logical Operator3 : Logic  Operator=NOT  IconShape=distinctive  AllPortsSameDT=off  OutDataTypeStr=boolean
  MATLAB Function1 : Subsystem
  ready : Outport  SampleTime=2.44140625e-07
  wires:
  advPop/1 -> Logical Operator1/1
  fifoCount/1 -> Generate Ready2/1(fifoCount)
  pop/1 -> Generate Ready2/2(pop)
  endReady/1 -> Logical Operator1/2
  Generate Ready2/1(ready2) -> Logical Operator2/1
  Logical Operator1/1 -> MATLAB Function1/1(trigger)
  Logical Operator2/1 -> ready/1
  Logical Operator3/1 -> Logical Operator2/2
  MATLAB Function1/1(out) -> Logical Operator3/1

== system gm_whdlOFDMTx/Frame Generator/Header/Interleaver/Read Logic ==
  fifoData : Inport  OutDataTypeStr=fixdt(0, 7, 0)  PortDimensions=1  SampleTime=2.44140625e-07
  fifoCount : Inport  Port=2  OutDataTypeStr=fixdt(0, 3, 0)  PortDimensions=1  SampleTime=2.44140625e-07
  Add1 : Sum  OutDataTypeStr=Inherit: Inherit via back propagation
  Delay1 : Delay  DelayLength=5
  Delay2 : Delay  DelayLength=5
  Delay3 : Delay  DelayLength=1
  Delay4 : Delay  DelayLength=5
  Delay7 : Delay  DelayLength=1
  Generate Base Read Address : Subsystem
  Generate Output Control Signals : Subsystem
  Generate Read Address : Subsystem
  MATLAB Function : Subsystem
  Relational Operator1 : RelationalOperator  Operator=<  OutDataTypeStr=boolean  InputSameDT=off
  Unit Delay Enabled Synchronous1 : hdlsllib/Discrete/Unit Delay Enabled Synchronous  InitialCondition=maxBlkSize -1  SampleTime=-1
  rdAddr : Outport  SampleTime=2.44140625e-07
  start : Outport  Port=2  SampleTime=2.44140625e-07
  end : Outport  Port=3  SampleTime=2.44140625e-07
  valid : Outport  Port=4  SampleTime=2.44140625e-07
  pop : Outport  Port=5  SampleTime=2.44140625e-07
  advPop : Outport  Port=6  SampleTime=2.44140625e-07
  wires:
  fifoData/1 -> Unit Delay Enabled Synchronous1/1
  fifoCount/1 -> Relational Operator1/1, Delay3/1
  Add1/1 -> Delay7/1
  Delay1/1 -> Add1/2
  Delay2/1 -> Generate Output Control Signals/2(blockValid)
  Delay3/1 -> Relational Operator1/2
  Delay4/1 -> Generate Output Control Signals/1(blockLen)
  Delay7/1 -> rdAddr/1
  Generate Base Read Address/1(baseAddr) -> Delay1/1
  Generate Output Control Signals/1(start) -> start/1
  Generate Output Control Signals/2(end) -> end/1
  Generate Output Control Signals/3(valid) -> valid/1
  Generate Output Control Signals/4(pop) -> pop/1
  Generate Output Control Signals/5(advPop) -> advPop/1
  Generate Read Address/1(blockDataCount) -> Generate Output Control Signals/3(blockCount)
  Generate Read Address/2(currentAddr) -> Add1/1
  MATLAB Function/1(out) -> Delay2/1, Generate Read Address/2(enable)
  Relational Operator1/1 -> Unit Delay Enabled Synchronous1/2, MATLAB Function/1(trigger), Generate Read Address/3(reset), Generate Base Read Address/1(readStart)
  Unit Delay Enabled Synchronous1/1 -> Delay4/1, Generate Read Address/1(blockLen)

== system gm_whdlOFDMTx/Frame Generator/Header/Interleaver/Write Logic ==
  start : Inport  OutDataTypeStr=boolean  PortDimensions=1  SampleTime=2.44140625e-07
  valid : Inport  Port=2  OutDataTypeStr=boolean  PortDimensions=1  SampleTime=2.44140625e-07
  end : Inport  Port=3  OutDataTypeStr=boolean  PortDimensions=1  SampleTime=2.44140625e-07
  Generate Write Address : Subsystem
  Handle Input Control Signals : Subsystem
  wrAddr : Outport  SampleTime=2.44140625e-07
  wrValid : Outport  Port=2  SampleTime=2.44140625e-07
  count : Outport  Port=3  SampleTime=2.44140625e-07
  endOut : Outport  Port=4  SampleTime=2.44140625e-07
  endReady : Outport  Port=5  SampleTime=2.44140625e-07
  wires:
  start/1 -> Handle Input Control Signals/1(start)
  valid/1 -> Handle Input Control Signals/2(valid)
  end/1 -> Handle Input Control Signals/3(end)
  Generate Write Address/1(wrAddr) -> wrAddr/1
  Generate Write Address/2(count) -> count/1
  Handle Input Control Signals/1(reset) -> Generate Write Address/1(rst)
  Handle Input Control Signals/2(countEnb) -> wrValid/1, Generate Write Address/2(enb)
  Handle Input Control Signals/3(endOut) -> endOut/1, Generate Write Address/3(end)
  Handle Input Control Signals/4(endReady) -> endReady/1

== system gm_whdlOFDMTx/Frame Generator/Header/Serializer/Serialize Start and End Signals ==
  startIn : Inport  OutDataTypeStr=boolean  PortDimensions=1  SampleTime=4.8828125e-07
  endIn : Inport  Port=2  OutDataTypeStr=boolean  PortDimensions=1  SampleTime=4.8828125e-07
  Delay : Delay  DelayLength=1
  Delay1 : Delay  DelayLength=1
  Delay2 : Delay  DelayLength=1
  Logical Operator : Logic  IconShape=distinctive  AllPortsSameDT=off  OutDataTypeStr=boolean
  Logical Operator1 : Logic  IconShape=distinctive  AllPortsSameDT=off  OutDataTypeStr=boolean
  Repeat : dspsigops/Repeat  N=length(headerConvCode)  RateOptions=Allow multirate processing  ic=0  mode=Unused parameter value
  Repeat1 : dspsigops/Repeat  N=length(headerConvCode)  RateOptions=Allow multirate processing  ic=0  mode=Unused parameter value
  startOut : Outport  SampleTime=2.44140625e-07
  endOut : Outport  Port=2  SampleTime=2.44140625e-07
  wires:
  startIn/1 -> Repeat/1
  endIn/1 -> Repeat1/1
  Delay/1 -> Logical Operator/2
  Delay1/1 -> Logical Operator1/2
  Delay2/1 -> endOut/1
  Logical Operator/1 -> startOut/1
  Logical Operator1/1 -> Delay2/1
  Repeat/1 -> Logical Operator/1, Delay/1
  Repeat1/1 -> Logical Operator1/1, Delay1/1

== system gm_whdlOFDMTx/Frame Controller and Input Sampler/Frame Controller/Generate OFDM Modulator Ready/Control OFDM Signal Generation/Disable OFDM Generation ==
  readyLow : Inport  OutDataTypeStr=boolean  PortDimensions=1  SampleTime=4.8828125e-07
  waitSignal : Inport  Port=2  OutDataTypeStr=boolean  PortDimensions=1  SampleTime=4.8828125e-07
  Delay3 : Delay  DelayLength=1
  Logical Operator12 : Logic  IconShape=distinctive  AllPortsSameDT=off  OutDataTypeStr=boolean
  Logical Operator13 : Logic  Operator=NOT  IconShape=distinctive  AllPortsSameDT=off  OutDataTypeStr=boolean
  MATLAB Function5 : Subsystem
  out : Outport  SampleTime=4.8828125e-07
  wires:
  readyLow/1 -> Logical Operator13/1
  waitSignal/1 -> Logical Operator12/2
  Delay3/1 -> MATLAB Function5/1(trigger)
  Logical Operator12/1 -> Delay3/1
  Logical Operator13/1 -> Logical Operator12/1
  MATLAB Function5/1(out) -> out/1

== system gm_whdlOFDMTx/Frame Controller and Input Sampler/Frame Controller/Generate OFDM Modulator Ready/Control OFDM Signal Generation/Falling Edge Detector ==
  in : Inport  OutDataTypeStr=boolean  PortDimensions=1  SampleTime=4.8828125e-07
  Delay3 : Delay  DelayLength=1
  Logical Operator1 : Logic  IconShape=distinctive  AllPortsSameDT=off  OutDataTypeStr=boolean
  Logical Operator2 : Logic  Operator=NOT  IconShape=distinctive  AllPortsSameDT=off  OutDataTypeStr=boolean
  out : Outport  SampleTime=4.8828125e-07
  wires:
  in/1 -> Logical Operator2/1, Delay3/1
  Delay3/1 -> Logical Operator1/1
  Logical Operator1/1 -> out/1
  Logical Operator2/1 -> Logical Operator1/2

== system gm_whdlOFDMTx/Frame Controller and Input Sampler/Frame Controller/Generate OFDM Modulator Ready/Control OFDM Signal Generation/MATLAB Function2 ==
  trigger : Inport  OutDataTypeStr=boolean  PortDimensions=1  SampleTime=4.8828125e-07
  MATLAB Function2 : MATLAB Function  TreatAsAtomicUnit=on  mask{nClocks=max(max(trBlkSize))}
      mask prompts: nClocks "Number of clocks to hold:"
  out : Outport  SampleTime=4.8828125e-07  VectorParamsAs1DForOutWhenUnconnected=off
  wires:
  trigger/1 -> MATLAB Function2/1(trigger)
  MATLAB Function2/1(out) -> out/1

== system gm_whdlOFDMTx/Frame Controller and Input Sampler/Frame Controller/Generate OFDM Modulator Ready/Control OFDM Signal Generation/Pulse Generator ==
  Constant : Constant  Value=true  SampleTime=-1
  Delay3 : Delay  DelayLength=1  InitialCondition=1
  Logical Operator3 : Logic  IconShape=distinctive  AllPortsSameDT=off  OutDataTypeStr=boolean
  Logical Operator4 : Logic  Operator=NOT  IconShape=distinctive  AllPortsSameDT=off  OutDataTypeStr=boolean
  pulse : Outport  SampleTime=4.8828125e-07
  wires:
  Constant/1 -> Logical Operator4/1, Logical Operator3/1
  Delay3/1 -> Logical Operator3/2
  Logical Operator3/1 -> pulse/1
  Logical Operator4/1 -> Delay3/1

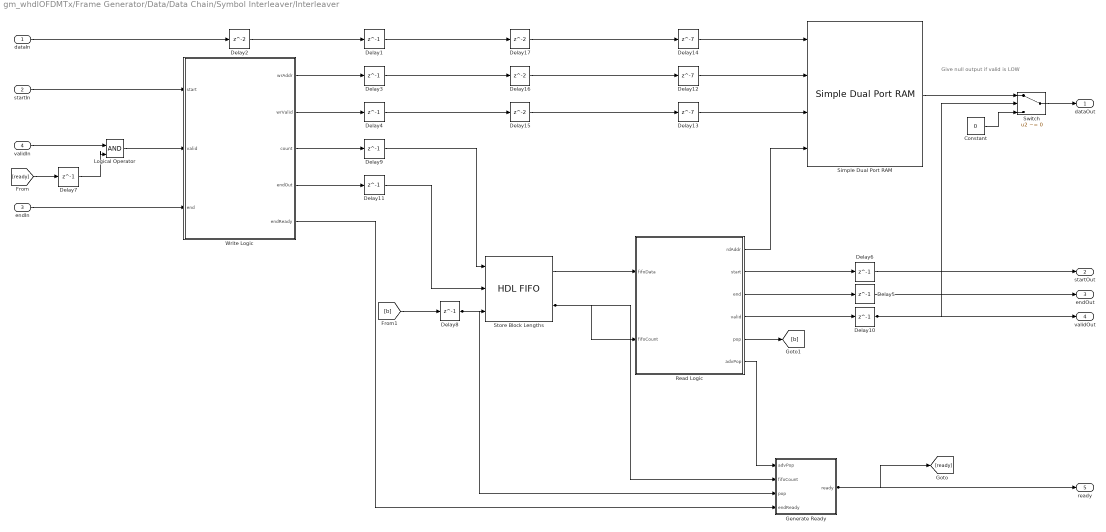
== system gm_whdlOFDMTx/Frame Generator/Data/Data Chain/Symbol Interleaver/Interleaver ==
  note: Give null output if valid is LOW
  dataIn : Inport  OutDataTypeStr=boolean  PortDimensions=1  SampleTime=2.44140625e-07
  startIn : Inport  Port=2  OutDataTypeStr=boolean  PortDimensions=1  SampleTime=2.44140625e-07
  endIn : Inport  Port=3  OutDataTypeStr=boolean  PortDimensions=1  SampleTime=2.44140625e-07
  validIn : Inport  Port=4  OutDataTypeStr=boolean  PortDimensions=1  SampleTime=2.44140625e-07
  Constant : Constant  Value=0  OutDataTypeStr=Inherit: Inherit via back propagation  SampleTime=-1
  Delay{1,3..6,9..11} (8 alike) : Delay  DelayLength=1
  Delay12 : Delay  DelayLength=7
  Delay13 : Delay  DelayLength=7
  Delay14 : Delay  DelayLength=7
  Delay{2,15..17} (4 alike) : Delay
  Delay7 : Delay  DelayLength=1  InitialCondition=true
  Delay8 : Delay  DelayLength=1  InitialCondition=true
  Generate Ready : Subsystem
  Logical Operator : Logic  IconShape=distinctive  AllPortsSameDT=off  OutDataTypeStr=boolean
  Read Logic : Subsystem
  Simple Dual Port RAM : hdlsllib/HDL RAMs/Simple Dual Port RAM  ram_size=nextpow2(2*maxBlkSize)
  Store Block Lengths : hdlsllib/HDL RAMs/HDL FIFO  fifo_size=4  mode=Classic  ratio=1  push_msg=Warning  pop_msg=Ignore  show_empty=off  show_full=off  show_num=on  LabelModeActiveChoice_Mode=Classic  rst_port=off
  Switch : Switch  Criteria=u2 ~= 0  SaturateOnIntegerOverflow=off
  Write Logic : Subsystem
  dataOut : Outport  SampleTime=2.44140625e-07
  startOut : Outport  Port=2  SampleTime=2.44140625e-07
  endOut : Outport  Port=3  SampleTime=2.44140625e-07
  validOut : Outport  Port=4  SampleTime=2.44140625e-07
  ready : Outport  Port=5  SampleTime=2.44140625e-07
  wires:
  dataIn/1 -> Delay2/1
  startIn/1 -> Write Logic/1(start)
  endIn/1 -> Write Logic/3(end)
  validIn/1 -> Logical Operator/1
  Constant/1 -> Switch/3
  Delay1/1 -> Delay17/1
  Delay10/1 -> Switch/2, validOut/1
  Delay11/1 -> Store Block Lengths/2
  Delay12/1 -> Simple Dual Port RAM/2
  Delay13/1 -> Simple Dual Port RAM/3
  Delay14/1 -> Simple Dual Port RAM/1
  Delay15/1 -> Delay13/1
  Delay16/1 -> Delay12/1
  Delay17/1 -> Delay14/1
  Delay2/1 -> Delay1/1
  Delay3/1 -> Delay16/1
  Delay4/1 -> Delay15/1
  Delay5/1 -> endOut/1
  Delay6/1 -> startOut/1
  Delay7/1 -> Logical Operator/2
  Delay8/1 -> Generate Ready/3(pop), Store Block Lengths/3
  Delay9/1 -> Store Block Lengths/1
  [ready] -> Delay7/1
  [b] -> Delay8/1
  Generate Ready/1(ready) -> [ready], ready/1
  Logical Operator/1 -> Write Logic/2(valid)
  Read Logic/1(rdAddr) -> Simple Dual Port RAM/4
  Read Logic/2(start) -> Delay6/1
  Read Logic/3(end) -> Delay5/1
  Read Logic/4(valid) -> Delay10/1
  Read Logic/5(pop) -> [b]
  Read Logic/6(advPop) -> Generate Ready/1(advPop)
  Simple Dual Port RAM/1 -> Switch/1
  Store Block Lengths/1 -> Read Logic/1(fifoData)
  Store Block Lengths/2 -> Generate Ready/2(fifoCount), Read Logic/2(fifoCount)
  Switch/1 -> dataOut/1
  Write Logic/1(wrAddr) -> Delay3/1
  Write Logic/2(wrValid) -> Delay4/1
  Write Logic/3(count) -> Delay9/1
  Write Logic/4(endOut) -> Delay11/1
  Write Logic/5(endReady) -> Generate Ready/4(endReady)

== system gm_whdlOFDMTx/Frame Generator/Data/Data Chain/Symbol Interleaver/Split Data Into Symbols ==
  data : Inport  OutDataTypeStr=boolean  PortDimensions=1  SampleTime=2.44140625e-07
  valid : Inport  Port=2  OutDataTypeStr=boolean  PortDimensions=1  SampleTime=2.44140625e-07
  modTypeIndex : Inport  Port=3  OutDataTypeStr=fixdt(0, 3, 0)  PortDimensions=1  SampleTime=2.44140625e-07
  Add : Sum  Inputs=+-  OutDataTypeStr=Inherit: Inherit via back propagation
  Compare To Constant : simulink/Logic and Bit Operations/Compare To Constant  relop===  const=0  OutDataTypeStr=boolean
  Constant : Constant  Value=(subC-(pilotLen/(NData)))*6  OutDataTypeStr=fixdt(0,nextpow2((subC-(pilotLen/(NData)))*6 +1),0)  SampleTime=-1
  Constant1 : Constant  Value=(subC-(pilotLen/(NData)))*4  OutDataTypeStr=fixdt(0,nextpow2((subC-(pilotLen/(NData)))*6 +1),0)  SampleTime=-1
  Constant2 : Constant  Value=(subC-(pilotLen/(NData)))*2  OutDataTypeStr=fixdt(0,nextpow2((subC-(pilotLen/(NData)))*6 +1),0)  SampleTime=-1
  Constant3 : Constant  Value=(subC-(pilotLen/(NData)))  OutDataTypeStr=fixdt(0,nextpow2((subC-(pilotLen/(NData)))*6 +1),0)  SampleTime=-1
  Constant4 : Constant  Value=2  OutDataTypeStr=fixdt(0,2,0)  SampleTime=-1
  Delay1 : Delay  DelayLength=1
  HDL Counter : hdlsllib/Sources/HDL Counter  CountType=Count limited  CountInit=0  CountStep=1  CountMax=(subC-(pilotLen/(NData)))*6 -1  CountFromType=Initial value  CountFrom=0  CountResetPort=on  CountLoadPort=off  CountEnbPort=on  CountDirPort=off  CountHitOutputPort=off  CountDataType=Unsigned  CountWordLen=nextpow2((subC-(pilotLen/(NData)))*6)  CountFracLen=0  CountSampTime=1
  Logical Operator : Logic  IconShape=distinctive  AllPortsSameDT=off  OutDataTypeStr=boolean
  Logical Operator1 : Logic  IconShape=distinctive  AllPortsSameDT=off  OutDataTypeStr=boolean
  Multiport Switch : MultiPortSwitch  DataPortOrder=Zero-based contiguous  Inputs=4  zeroidx=on  SaturateOnIntegerOverflow=off  InputSameDT=off
  Relational Operator : RelationalOperator  Operator===  OutDataTypeStr=boolean  InputSameDT=off
  dataOut : Outport  SampleTime=2.44140625e-07
  startOut : Outport  Port=2  SampleTime=2.44140625e-07
  endOut : Outport  Port=3  SampleTime=2.44140625e-07
  validOut : Outport  Port=4  SampleTime=2.44140625e-07
  wires:
  data/1 -> dataOut/1
  valid/1 -> Logical Operator1/2, Logical Operator/2, validOut/1, HDL Counter/2
  modTypeIndex/1 -> Multiport Switch/1
  Add/1 -> Relational Operator/1
  Compare To Constant/1 -> Logical Operator/1
  Constant/1 -> Multiport Switch/5
  Constant1/1 -> Multiport Switch/4
  Constant2/1 -> Multiport Switch/3
  Constant3/1 -> Multiport Switch/2
  Constant4/1 -> Add/2
  Delay1/1 -> endOut/1, HDL Counter/1
  HDL Counter/1 -> Relational Operator/2, Compare To Constant/1
  Logical Operator/1 -> startOut/1
  Logical Operator1/1 -> Delay1/1
  Multiport Switch/1 -> Add/1
  Relational Operator/1 -> Logical Operator1/1

== system gm_whdlOFDMTx/Frame Generator/Header/Interleaver/Generate Ready/Generate Ready2 ==
  fifoCount : Inport  OutDataTypeStr=fixdt(0, 3, 0)  PortDimensions=1  SampleTime=2.44140625e-07
  pop : Inport  Port=2  OutDataTypeStr=boolean  PortDimensions=1  SampleTime=2.44140625e-07
  Compare To Constant1 : simulink/Logic and Bit Operations/Compare To Constant  relop===  const=0  OutDataTypeStr=boolean
  Compare To Constant4 : simulink/Logic and Bit Operations/Compare To Constant  relop===  const=1  OutDataTypeStr=boolean
  Logical Operator1 : Logic  Operator=OR  IconShape=distinctive  AllPortsSameDT=off  OutDataTypeStr=boolean
  Logical Operator14 : Logic  IconShape=distinctive  AllPortsSameDT=off  OutDataTypeStr=boolean
  ready2 : Outport  SampleTime=2.44140625e-07
  wires:
  fifoCount/1 -> Compare To Constant4/1, Compare To Constant1/1
  pop/1 -> Logical Operator14/2
  Compare To Constant1/1 -> Logical Operator1/1
  Compare To Constant4/1 -> Logical Operator14/1
  Logical Operator1/1 -> ready2/1
  Logical Operator14/1 -> Logical Operator1/2

== system gm_whdlOFDMTx/Frame Generator/Header/Interleaver/Generate Ready/MATLAB Function1 ==
  trigger : Inport  OutDataTypeStr=boolean  PortDimensions=1  SampleTime=2.44140625e-07
  MATLAB Function1 : MATLAB Function  TreatAsAtomicUnit=on  mask{nClocks=4}
      mask prompts: nClocks "Number of clocks to hold:"
  out : Outport  SampleTime=2.44140625e-07  VectorParamsAs1DForOutWhenUnconnected=off
  wires:
  trigger/1 -> MATLAB Function1/1(trigger)
  MATLAB Function1/1(out) -> out/1
